simulink model "sub_multicore"  (R2017a)
settings: Solver=VariableStepAuto  StartTime=0.0  StopTime=10.0  RelTol=1e-3
libraries: sharedutil x2
settings Model: Creator=hp  LastModifiedBy=hp

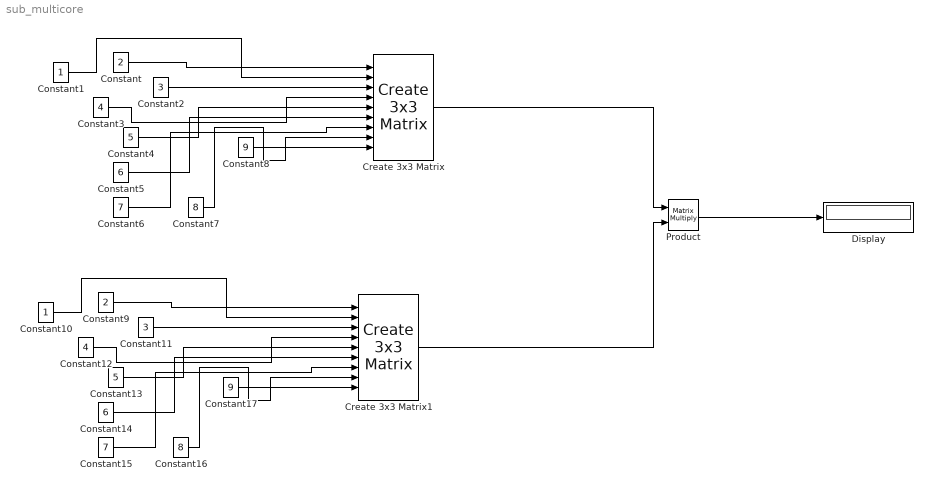
== system sub_multicore ==
  Constant : Constant  Value=2
  Constant1 : Constant
  Constant10 : Constant
  Constant11 : Constant  Value=3
  Constant12 : Constant  Value=4
  Constant13 : Constant  Value=5
  Constant14 : Constant  Value=6
  Constant15 : Constant  Value=7
  Constant16 : Constant  Value=8
  Constant17 : Constant  Value=9
  Constant2 : Constant  Value=3
  Constant3 : Constant  Value=4
  Constant4 : Constant  Value=5
  Constant5 : Constant  Value=6
  Constant6 : Constant  Value=7
  Constant7 : Constant  Value=8
  Constant8 : Constant  Value=9
  Constant9 : Constant  Value=2
  Create 3x3 Matrix : sharedutil/Create 3x3 Matrix
  Create 3x3 Matrix1 : sharedutil/Create 3x3 Matrix
  Display : Display
  Product : Product  Multiplication=Matrix(*)
  wires:
  Constant2/1 -> Create 3x3 Matrix/3
  Constant3/1 -> Create 3x3 Matrix/4
  Constant7/1 -> Create 3x3 Matrix/8
  Constant1/1 -> Create 3x3 Matrix/2
  Constant8/1 -> Create 3x3 Matrix/9
  Create 3x3 Matrix/1 -> Product/1
  Constant4/1 -> Create 3x3 Matrix/5
  Constant/1 -> Create 3x3 Matrix/1
  Constant6/1 -> Create 3x3 Matrix/7
  Constant5/1 -> Create 3x3 Matrix/6
  Create 3x3 Matrix1/1 -> Product/2
  Constant13/1 -> Create 3x3 Matrix1/5
  Constant14/1 -> Create 3x3 Matrix1/6
  Constant12/1 -> Create 3x3 Matrix1/4
  Constant9/1 -> Create 3x3 Matrix1/1
  Constant15/1 -> Create 3x3 Matrix1/7
  Constant17/1 -> Create 3x3 Matrix1/9
  Constant11/1 -> Create 3x3 Matrix1/3
  Constant16/1 -> Create 3x3 Matrix1/8
  Constant10/1 -> Create 3x3 Matrix1/2
  Product/1 -> Display/1
